simulink model "UDP_Sender"  (R2023b)
settings: Solver=ode4  StartTime=0.0  StopTime=inf  FixedStep=1/100  RelTol=1e-3
libraries: dspnetwork x1
settings Model: SimulationMode=accelerator  Creator=MONSTER  LastModifiedBy=MONSTER

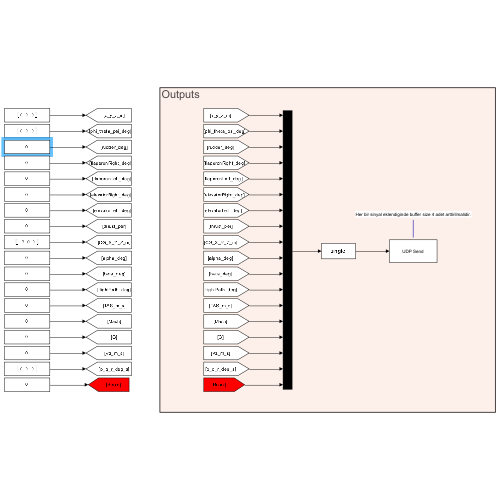
[thumbnail: Simulink's stored preview of the top-level diagram]
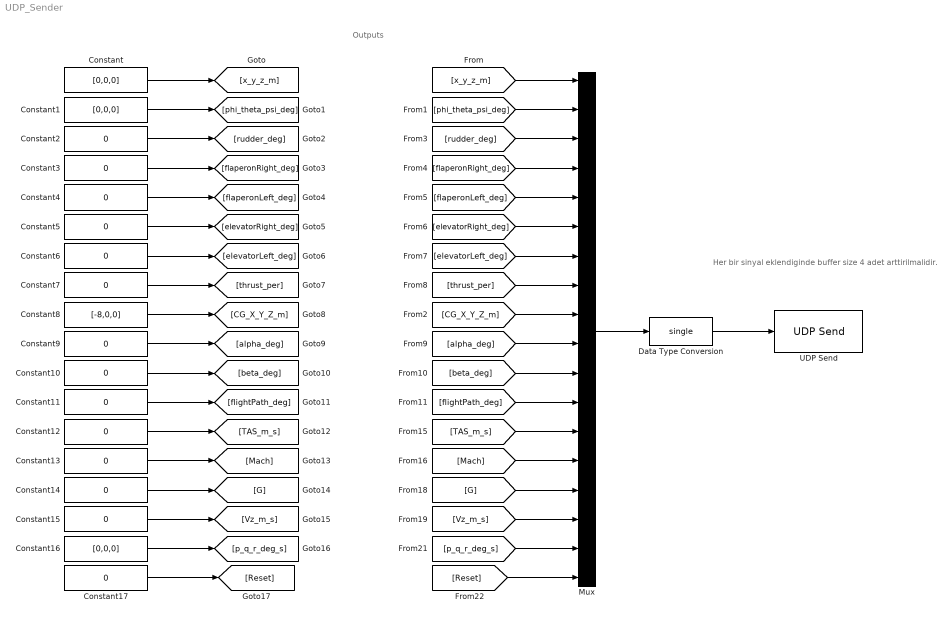
== system UDP_Sender ==
  note: Her bir sinyal eklendiginde buffer size 4 adet arttirilmalidir.
  note: Outputs
  Constant : Constant  Value=[0,0,0]
  Constant1 : Constant  Value=[0,0,0]
  Constant{2..7,9..15,17} (14 alike) : Constant  Value=0
  Constant16 : Constant  Value=[0,0,0]
  Constant8 : Constant  Value=[-8,0,0]
  Data Type Conversion : DataTypeConversion  OutDataTypeStr=single  SaturateOnIntegerOverflow=off  RndMeth=Floor
  Mux : Mux  Inputs=18
  UDP Send : dspnetwork/UDP Send  remoteURL='127.0.0.1'  remotePort=8001  localURL='0.0.0.0'  localPortSource=Automatically determine  localPort=-1  sendBufferSize=104  sampletime=-1  blockPlatform=[]  separateLengthPort=0
  wires:
  [beta_deg] -> Mux/11
  [TAS_m_s] -> Mux/13
  [Reset] -> Mux/18
  [flightPath_deg] -> Mux/12
  [thrust_per] -> Mux/8
  [elevatorRight_deg] -> Mux/6
  [flaperonLeft_deg] -> Mux/5
  Mux/1 -> Data Type Conversion/1
  [phi_theta_psi_deg] -> Mux/2
  Data Type Conversion/1 -> UDP Send/1
  [p_q_r_deg_s] -> Mux/17
  [elevatorLeft_deg] -> Mux/7
  [rudder_deg] -> Mux/3
  [flaperonRight_deg] -> Mux/4
  [G] -> Mux/15
  [Mach] -> Mux/14
  [Vz_m_s] -> Mux/16
  [x_y_z_m] -> Mux/1
  [alpha_deg] -> Mux/10
  [CG_X_Y_Z_m] -> Mux/9
  Constant/1 -> [x_y_z_m]
  Constant1/1 -> [phi_theta_psi_deg]
  Constant2/1 -> [rudder_deg]
  Constant3/1 -> [flaperonRight_deg]
  Constant4/1 -> [flaperonLeft_deg]
  Constant5/1 -> [elevatorRight_deg]
  Constant6/1 -> [elevatorLeft_deg]
  Constant7/1 -> [thrust_per]
  Constant8/1 -> [CG_X_Y_Z_m]
  Constant9/1 -> [alpha_deg]
  Constant10/1 -> [beta_deg]
  Constant11/1 -> [flightPath_deg]
  Constant12/1 -> [TAS_m_s]
  Constant13/1 -> [Mach]
  Constant14/1 -> [G]
  Constant15/1 -> [Vz_m_s]
  Constant16/1 -> [p_q_r_deg_s]
  Constant17/1 -> [Reset]
